simulink model "main"  (R2021a)
settings: Solver=ode113  StartTime=0.0  StopTime=300  RelTol=1e-13  AbsTol=1e-14
values from neighbouring files (symbols this model uses):
  Const = createSimulinkBus(Const_1)    [initializeData.m]
  Earth = createSimulinkBus(Earth_1)    [initializeData.m]
  Sensors = createSimulinkBus(Sensors_1)    [initializeData.m]
  Spacecraft = createSimulinkBus(Spacecraft_1)    [initializeData.m]
  totalTorque = [0 0 0 0.000704944678681 0.000834848489248 0.000628617928475 0.000704944678681 -0.000834848489248 -0.000628617928475 0.00140988935736 0 0 ... (48 elements, 3x16)]    [totalTorque.mat]
undefined symbols (not defined in the file or in its folder): initCond, torqueLookUpTable
libraries: simulink x22, SADlibrary x22, aerolibutil x20, vrlib x14, dspsrcs4 x12, sharedtransform x5, commfilt2 x3, dspfdesign x3, simulink_extras x2, sharedTrackingLibrary x2, dspmathops x1, sharedutil x1
(part 1 of 2)
settings Model: SimulationMode=rapid-accelerator  Creator=matteo  LastModifiedBy=matteo
settings SolverCC: ZeroCrossControl=EnableAll  ZeroCrossAlgorithm=Adaptive  AlgebraicLoopSolver=TrustRegion  DecoupledContinuousIntegration=on
settings DebuggingCC: ReadBeforeWriteMsg=DisableAll  WriteAfterWriteMsg=DisableAll  WriteAfterReadMsg=DisableAll  MultiTaskDSMMsg=none  SFMachineParentedDataDiag=warning
settings ModelReferenceCC: UpdateModelReferenceTargets=IfOutOfDate
settings SFSimCC: SFSimEcho=off
settings SimscapeCC: SimscapeNormalizeSystem=off

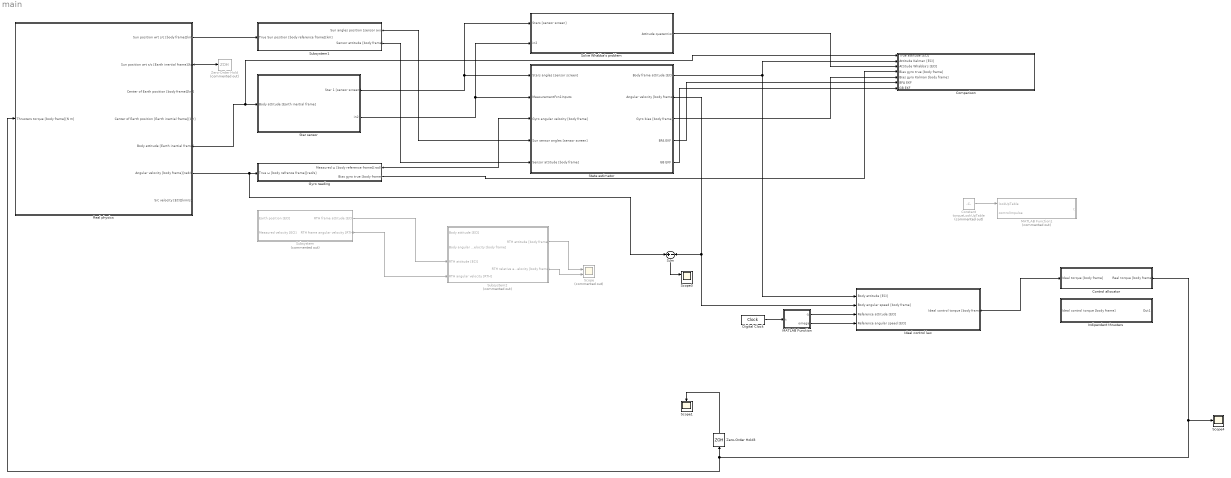
== system main ==
  Comparison : Subsystem
  Constant : Constant  Commented=on  Value=torqueLookUpTable
  Control allocator : Subsystem
  Digital Clock : DigitalClock  SampleTime=1/1000
  Gyro reading : Subsystem
  Ideal control law : Subsystem
  Indipendent thrusters : Subsystem
  MATLAB Function : MATLAB Function  TreatAsAtomicUnit=on
  MATLAB Function1 : MATLAB Function  Commented=on  TreatAsAtomicUnit=on
  Real physics : Subsystem
  Scope : Scope  Commented=on  NumInputPorts=2
  Scope1 : Scope
  Scope3 : Scope  NumInputPorts=2
  Scope4 : Scope
  Solve Whabba's problem : Subsystem
  Star sensor : Subsystem
  State estimator : Subsystem
  Subsystem : Subsystem  Commented=on
  Subsystem1 : Subsystem
  Subsystem2 : Subsystem  Commented=on
  Sum : Sum  Inputs=+-
  Zero-Order Hold : ZeroOrderHold  Commented=on  SampleTime=Sensors.sunSensorSamplingFreq
  Zero-Order Hold3 : ZeroOrderHold  SampleTime=.01
  wires:
  Real physics/6(Angular velocity [body frame][rad/s]) -> Sum/1, Gyro reading/1(True ω [body refrence frame][rad/s])
  Real physics/2(Sun position wrt s/c [Earth inertial frame][km]) -> Zero-Order Hold/1
  Real physics/1(Sun position wrt s/c [body frame][km]) -> Subsystem1/1(True Sun position [body reference frame][km])
  Subsystem/1(RTH frame attitude [ECI]) -> Subsystem2/3(RTH attitude [ECI])
  Subsystem/2("RTH frame angular velocity [RTH] ") -> Subsystem2/4(RTH angular velocity [RTH])
  Subsystem2/1(RTH attitude [body frame]) -> Scope/1
  Subsystem2/2(RTH relative angular velocity [body frame]) -> Scope/2
  Zero-Order Hold3/1 -> Scope1/1
  Real physics/5(Body attitude [Earth inertial frame]) -> Comparison/1(True attitude [ECI]), Star sensor/1(Body attitude [Earth inertial frame])
  Star sensor/1(Star 1 [sensor screen]) -> Solve Whabba's problem/1(Stars [sensor screen]), State estimator/1(Stars angles [sensor screen])
  Star sensor/2(in2) -> State estimator/2(MeasurementFcn1Inputs), Solve Whabba's problem/2(in2)
  Gyro reading/1(Measured ω [body reference frame][rad/s]) -> State estimator/3(Gyro angular velocity [body frame])
  State estimator/1(Body frame attitude [ECI]) -> Ideal control law/1(Body attitude [ECI]), Comparison/2(Attitude Kalman [ECI])
  Solve Whabba's problem/1(Attitude quaternion) -> Comparison/3(Attitude Whabba's [ECI])
  State estimator/2(Angular velocity [body frame]) -> Sum/2, Ideal control law/2(Body angular speed [body frame])
  Gyro reading/2(Bias gyro true [body frame]) -> Comparison/4(Bias gyro true [body frame])
  State estimator/3(Gyro bias [body frame]) -> Comparison/5(Bias gyro Kalman [body frame])
  Sum/1 -> Scope3/1
  MATLAB Function/1(q) -> Ideal control law/3(Reference attitude [ECI])
  MATLAB Function/2(omega) -> Ideal control law/4(Reference angular speed [ECI])
  State estimator/4(BFA EKF) -> Comparison/6(BFA EKF)
  State estimator/5(GB EKF) -> Comparison/7(GB EKF)
  Constant/1 -> MATLAB Function1/1(lookUpTable)
  Digital Clock/1 -> MATLAB Function/1(t)
  Control allocator/1(Real torque [body frame]) -> Real physics/1(Thrusters torque [body frame][N m]), Zero-Order Hold3/1, Scope4/1
  Subsystem1/1(Sun angles position [sensor axis]) -> State estimator/4(Sun sensor angles [sensor screen])
  Subsystem1/2(Sensor attitude [body frame]) -> State estimator/5(Sensor attitude [body frame])
  Ideal control law/1(Ideal control torque [body frame]) -> Control allocator/1(Ideal torque [body frame])

== system main/Comparison ==
  True attitude [ECI] : Inport
  Attitude Kalman [ECI] : Inport  Port=2
  Attitude Whabba's [ECI] : Inport  Port=3
  Bias gyro true [body frame] : Inport  Port=4
  Bias gyro Kalman [body frame] : Inport  Port=5
  BFA EKF : Inport  Port=6
  GB EKF : Inport  Port=7
  MATLAB Function : MATLAB Function  TreatAsAtomicUnit=on
  MATLAB Function1 : MATLAB Function  TreatAsAtomicUnit=on
  MATLAB Function2 : MATLAB Function  TreatAsAtomicUnit=on
  Quaternion Division1 : aerolibutil/Quaternion Division
      settings: SourceProductBaseCode=AE
  Quaternion Division2 : aerolibutil/Quaternion Division
      settings: SourceProductBaseCode=AE
  Quaternion Division3 : aerolibutil/Quaternion Division
      settings: SourceProductBaseCode=AE
  Scope : Scope  NumInputPorts=3
  Scope1 : Scope  NumInputPorts=3
  wires:
  True attitude [ECI]/1 -> Quaternion Division3/1, Quaternion Division1/1, Quaternion Division2/1
  Attitude Kalman [ECI]/1 -> Quaternion Division2/2
  Attitude Whabba's [ECI]/1 -> Quaternion Division1/2
  Quaternion Division2/1 -> MATLAB Function1/1(q)  "Kalman error"
  Bias gyro true [body frame]/1 -> Scope1/1
  Bias gyro Kalman [body frame]/1 -> Scope1/2
  MATLAB Function1/1(e) -> Scope/1  "Kalman error"
  MATLAB Function/1(e) -> Scope/2  "Whabba's error"
  Quaternion Division1/1 -> MATLAB Function/1(q)  "Whabba's error"
  BFA EKF/1 -> Quaternion Division3/2
  Quaternion Division3/1 -> MATLAB Function2/1(q)  "Whabba's error"
  MATLAB Function2/1(e) -> Scope/3  "Whabba's error"
  GB EKF/1 -> Scope1/3

== system main/Control allocator ==
  Ideal torque [body frame] : Inport
  Constant1 : Constant  Value=thrustersTorque'  VectorParams1D=off
  Demux3 : Demux  Outputs=3
  Gain18 : Gain
  Gain19 : Gain
  Gain5 : Gain  Gain=1/2
  Integrate and Dump4 : commfilt2/Integrate and Dump  obssamples=200  offsetsamples=0  nodump=off  roundingMode=Floor  overflowMode=off  outputDataTypeStr=Inherit: Same as accumulator  outputLastDataTypeStr=Inherit: Same as accumulator
  Integrate and Dump5 : commfilt2/Integrate and Dump  obssamples=200  offsetsamples=0  nodump=off  roundingMode=Floor  overflowMode=off  outputDataTypeStr=Inherit: Same as accumulator  outputLastDataTypeStr=Inherit: Same as accumulator
  Integrate and Dump6 : commfilt2/Integrate and Dump  obssamples=200  offsetsamples=0  nodump=off  roundingMode=Floor  overflowMode=off  outputDataTypeStr=Inherit: Same as accumulator  outputLastDataTypeStr=Inherit: Same as accumulator
  MATLAB Function3 : MATLAB Function  TreatAsAtomicUnit=on
  Mux2 : Mux  Inputs=3
  Subsystem3 : Subsystem
  Real torque [body frame] : Outport
  wires:
  Gain19/1 -> Real torque [body frame]/1
  Gain18/1 -> MATLAB Function3/1(cgtTorque)
  Integrate and Dump6/1 -> Mux2/1
  Demux3/2 -> Integrate and Dump4/1
  Gain5/1 -> MATLAB Function3/2(dGammaId)
  Constant1/1 -> Gain18/1
  MATLAB Function3/1(xOpt) -> Subsystem3/1(uTimes)
  Demux3/1 -> Integrate and Dump6/1
  Demux3/3 -> Integrate and Dump5/1
  Subsystem3/1(Real torque) -> Gain19/1
  Mux2/1 -> Gain5/1
  Integrate and Dump4/1 -> Mux2/2
  Ideal torque [body frame]/1 -> Demux3/1
  Integrate and Dump5/1 -> Mux2/3

== system main/Gyro reading ==
  True ω [body refrence frame][rad/s] : Inport
  Constant : Constant  Value=1e-3*randn(3,1)
  Cumulative Sum : dspmathops/Cumulative Sum  dim=Channels (running sum)  reset_popup=None  roundingMode=Floor  overflowMode=off  outputDataTypeStr=Inherit: Same as accumulator  outputMin=[]  outputMax=[]  outputLastDataTypeStr=Inherit: Same as accumulator
  Gain : Gain  Gain=sqrt(1/Sensors.gyroSamplingFreq)
  Random Source : dspsrcs4/Random Source  SrcType=Gaussian  NormMethod=Ziggurat  CltLength=12  MinVal=0  MaxVal=1  MeanVal=0  VarVal=Sensors.gyroCovariance  RepMode=Not repeatable  rawSeed=1  IsInherit=off  SampMode=Discrete  SampTime=1/Sensors.gyroSamplingFreq  SampFrame=3  DataType=Double  OutComplex=Real  OutputFrames=off
  Random Source1 : dspsrcs4/Random Source  SrcType=Gaussian  NormMethod=Ziggurat  CltLength=12  MinVal=0  MaxVal=1  MeanVal=0  VarVal=Sensors.gyroBiasInstability  RepMode=Not repeatable  rawSeed=1  IsInherit=off  SampMode=Discrete  SampTime=1/Sensors.gyroSamplingFreq  SampFrame=3  DataType=Double  OutComplex=Real  OutputFrames=off
  Sum : Sum  Inputs=|++
  Sum1 : Sum  Inputs=|++
  Sum2 : Sum  Inputs=|++
  Zero-Order Hold : ZeroOrderHold  SampleTime=1/Sensors.gyroSamplingFreq
  Measured ω [body reference frame][rad/s] : Outport
  Bias gyro true [body frame] : Outport  Port=2
  wires:
  Sum2/1 -> Measured ω [body reference frame][rad/s]/1
  True ω [body refrence frame][rad/s]/1 -> Zero-Order Hold/1
  Cumulative Sum/1 -> Sum1/2
  Gain/1 -> Cumulative Sum/1
  Random Source1/1 -> Gain/1
  Constant/1 -> Sum1/1
  Zero-Order Hold/1 -> Sum/1
  Random Source/1 -> Sum/2
  Sum/1 -> Sum2/1
  Sum1/1 -> Bias gyro true [body frame]/1, Sum2/2

== system main/Ideal control law ==
  note: $q_e := q_{B/R} = q_{B/N} \otimes q_{R/N}^{-1}$
  Body attitude [ECI] : Inport
  Body angular speed [body frame] : Inport  Port=2
  Reference attitude [ECI] : Inport  Port=3
  Reference angular speed [ECI] : Inport  Port=4
  Constant : Constant  Value=Spacecraft.baricentricInertia
  Constant1 : Constant  Value=totalTorque
  MATLAB Function : MATLAB Function  TreatAsAtomicUnit=on
  MATLAB Function1 : MATLAB Function  TreatAsAtomicUnit=on
  MATLAB Function2 : MATLAB Function  TreatAsAtomicUnit=on
  Quaternion Division : aerolibutil/Quaternion Division
      settings: SourceProductBaseCode=AE
  Quaternion Rotation : aerolibutil/Quaternion Rotation
  Scope : Scope  NumInputPorts=4
  Scope1 : Scope
  Scope2 : Scope
  Sum : Sum  Inputs=|+-
  Ideal control torque [body frame] : Outport
  wires:
  Quaternion Division/1 -> MATLAB Function1/1(q), MATLAB Function2/5(qErr), MATLAB Function/4(qErr), Scope/1  "Attitude error"
  Reference angular speed [ECI]/1 -> Quaternion Rotation/2
  Quaternion Rotation/1 -> Sum/2  "Reference angular speed [body frame]"
  Body angular speed [body frame]/1 -> MATLAB Function2/3(omegaBody), MATLAB Function/2(omegaBody), Sum/1
  Sum/1 -> Scope1/1, MATLAB Function2/4(omegaErr), MATLAB Function/3(omegaErr)  "Angular speed error [body frame]"
  Constant/1 -> MATLAB Function/1(J), MATLAB Function2/1(J)
  Reference attitude [ECI]/1 -> Scope/4, Quaternion Division/2
  Body attitude [ECI]/1 -> Scope/3, Quaternion Division/1, Quaternion Rotation/1
  MATLAB Function1/1(e) -> Scope/2
  Constant1/1 -> MATLAB Function2/2(torque)
  MATLAB Function2/2(VdotMin) -> Scope2/1
  MATLAB Function/1(u) -> Ideal control torque [body frame]/1

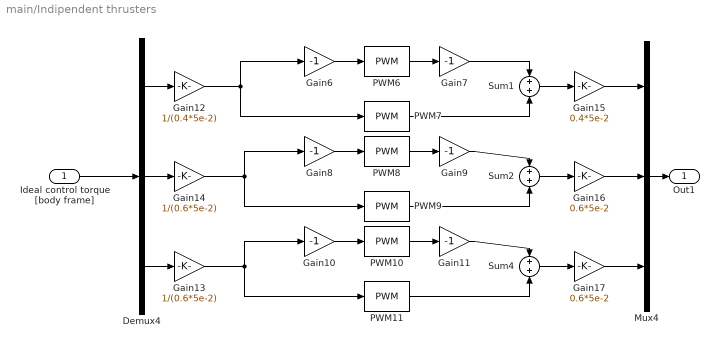
== system main/Indipendent thrusters ==
  Ideal control torque [body frame] : Inport
  Demux4 : Demux  Outputs=3
  Gain{6..11} (6 alike) : Gain  Gain=-1
  Gain12 : Gain  Gain=1/(0.4*5e-2)
  Gain13 : Gain  Gain=1/(0.6*5e-2)
  Gain14 : Gain  Gain=1/(0.6*5e-2)
  Gain15 : Gain  Gain=0.4*5e-2
  Gain16 : Gain  Gain=0.6*5e-2
  Gain17 : Gain  Gain=0.6*5e-2
  Mux4 : Mux  Inputs=3
  PWM{6..11} (6 alike) : simulink/Discontinuities/PWM  DisableCoverage=on  Period=0.5  DisallowZeroDutyCycle=off  RunAtFixedTimeIntervals=on  SampleTime=1/Sensors.gyroSamplingFreq
  Sum1 : Sum
  Sum2 : Sum
  Sum4 : Sum
  Out1 : Outport
  wires:
  PWM8/1 -> Gain9/1
  Mux4/1 -> Out1/1
  PWM11/1 -> Sum4/2
  Gain11/1 -> Sum4/1
  PWM6/1 -> Gain7/1
  Sum2/1 -> Gain16/1
  PWM10/1 -> Gain11/1
  Gain12/1 -> PWM7/1, Gain6/1
  Gain17/1 -> Mux4/3
  PWM7/1 -> Sum1/2
  Gain6/1 -> PWM6/1
  Gain16/1 -> Mux4/2
  Gain9/1 -> Sum2/1
  Gain14/1 -> PWM9/1, Gain8/1
  Demux4/1 -> Gain12/1
  Gain10/1 -> PWM10/1
  Gain13/1 -> PWM11/1, Gain10/1
  Demux4/2 -> Gain14/1
  Sum4/1 -> Gain17/1
  Ideal control torque [body frame]/1 -> Demux4/1
  Sum1/1 -> Gain15/1
  Gain8/1 -> PWM8/1
  Gain15/1 -> Mux4/1
  Demux4/3 -> Gain13/1
  PWM9/1 -> Sum2/2
  Gain7/1 -> Sum1/1

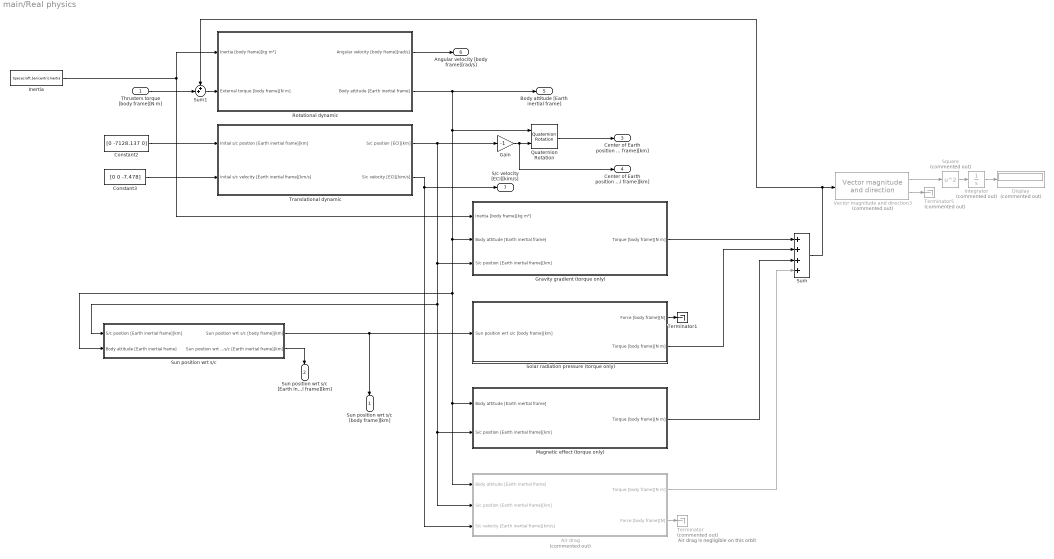
== system main/Real physics ==
  note: Air drag is negligible on this orbit
  Thrusters torque [body frame][N m] : Inport  Unit=N*m
  Air drag : Subsystem  Commented=on
  Constant2 : Constant  Value=[0 -7128.137 0]
  Constant3 : Constant  Value=[0 0 -7.478]
  Display : Display  Commented=on
  Gain : Gain  Gain=-1
  Gravity gradient (torque only) : Subsystem
      settings: PortSchema="{\"entries\":[{\"content\":{\"sides\":[{\"content\":{\"connectorIds\":[\"Out1\"]},\"type\":\"ConnectorPlacement.EquallySpacedRectSide\",\"uuid\":\"f1f9fb06-69b8-4265-b1e3-1bc99765f445\"},{\"content\":{\"connectorIds\":[\"In1\",\"In2\",\"In3\"],\"side\":\"RIGHT\"},\"type\":\"ConnectorPlacement.EquallySpacedRectSide\",\"uuid\":\"95872401-8fe8-493a-a743-72ee2e043305\"},{\"content\":{\"connectorIds\":[],\"side\":\"TOP\"},\"type\":\"ConnectorPlacement.EquallySpacedRectSide\",\"uuid\":\"a2f933f3-d116-4556-b216-8e543aff18f5\"},{\"content\":{\"connectorIds\":[],\"side\":\"HIDDEN\"},\"type\":\"ConnectorPlacement.EquallySpacedRectSide\",\"uuid\":\"93d45030-e624-494e-a335-b0ea445a7c18\"}]},\"type\":\"ConnectorPlacement.EquallySpacedConnector\",\"uuid\":\"bbb7bc93-29be-48e8-9ed7-f6b41cc2b7e1\"}],\"packageUris\":[\"http://schema.mathworks.com/mf0/Connector/R2020b\"],\"version\":\"1.0\"}"
  Inertia : Constant  Value=Spacecraft.baricentricInertia
  Integrator : Integrator  Commented=on
  Magnetic effect (torque only) : Subsystem
  Quaternion Rotation : aerolibutil/Quaternion Rotation
  Rotational dynamic : Subsystem
  Solar radiation pressure (torque only) : Subsystem
  Square : Math  Commented=on  Operator=square  SaturateOnIntegerOverflow=on
  Sum : Sum  Inputs=++++
  Sum1 : Sum  Inputs=++|
  Sun position wrt s/c : Subsystem
  Terminator : Terminator  Commented=on
  Terminator1 : Terminator
  Terminator5 : Terminator  Commented=on
  Translational dynamic : Subsystem
  Vector magnitude and direction3 : SADlibrary/Vector magnitude and direction  Commented=on  SystemSampleTime=-1  VariantActivationTime=update diagram  Latency=0  AutoFrameSizeCalculation=off
  Sun position wrt s/c [body frame][km] : Outport  OutDataTypeStr=double  Unit=km
  Sun position wrt s/c [Earth inertial frame][km] : Outport  Port=2
  Center of Earth position [body frame][km] : Outport  Port=3
  Center of Earth position [Earth inertial frame][km] : Outport  Port=4
  Body attitude [Earth inertial frame] : Outport  Port=5
  Angular velocity [body frame][rad/s] : Outport  Port=6
  S/c velocity [ECI][kim/s] : Outport  Port=7
  wires:
  Inertia/1 -> Gravity gradient (torque only)/1(Inertia [body frame][kg m²]), Rotational dynamic/1(Inertia [body frame][kg m²])
  Rotational dynamic/1(Angular velocity [body frame][rad/s]) -> Angular velocity [body frame][rad/s]/1
  Constant2/1 -> Translational dynamic/1(Initial s/c position [Earth inertial frame][km])
  Constant3/1 -> Translational dynamic/2(Initial s/c velocity [Earth inertial frame][km/s])
  Rotational dynamic/2(Body attitude [Earth inertial frame]) -> Body attitude [Earth inertial frame]/1, Quaternion Rotation/1, Air drag/1(Body attitude [Earth inertial frame]), Magnetic effect (torque only)/1(Body attitude [Earth inertial frame]), Sun position wrt s/c/2(Body attitude [Earth inertial frame]), Gravity gradient (torque only)/2(Body attitude [Earth inertial frame])
  Translational dynamic/1(S/c position [ECI][km]) -> Gain/1, Gravity gradient (torque only)/3(S/c position [Earth inertial frame][km]), Sun position wrt s/c/1(S/c position [Earth inertial frame][km]), Air drag/2(S/c position [Earth inertial frame][km]), Magnetic effect (torque only)/2(S/c position [Earth inertial frame][km])
  Sum/1 -> Sum1/1, Vector magnitude and direction3/1
  Air drag/2(Force [body frame][N]) -> Terminator/1
  Solar radiation pressure (torque only)/1(Force [body frame][N]) -> Terminator1/1
  Sun position wrt s/c/1(Sun position wrt s/c [body frame][km]) -> Solar radiation pressure (torque only)/1(Sun position wrt s/c [body frame][km]), Sun position wrt s/c [body frame][km]/1
  Solar radiation pressure (torque only)/2(Torque [body frame][N m]) -> Sum/2
  Magnetic effect (torque only)/1(Torque [body frame][N m]) -> Sum/3
  Air drag/1(Torque [body frame][N m]) -> Sum/4
  Gravity gradient (torque only)/1(Torque [body frame][N m]) -> Sum/1
  Gain/1 -> Center of Earth position [Earth inertial frame][km]/1, Quaternion Rotation/2
  Quaternion Rotation/1 -> Center of Earth position [body frame][km]/1
  Sun position wrt s/c/2(Sun position wrt s/c [Earth inertial frame][km]) -> Sun position wrt s/c [Earth inertial frame][km]/1
  Thrusters torque [body frame][N m]/1 -> Sum1/2
  Sum1/1 -> Rotational dynamic/2(External torque [body frame][N m])
  Vector magnitude and direction3/1 -> Square/1
  Vector magnitude and direction3/2 -> Terminator5/1
  Square/1 -> Integrator/1
  Integrator/1 -> Display/1
  Translational dynamic/2(S/c velocity [ECI][kim/s]) -> S/c velocity [ECI][kim/s]/1, Air drag/3(S/c velocity [Earth inertial frame][km/s])

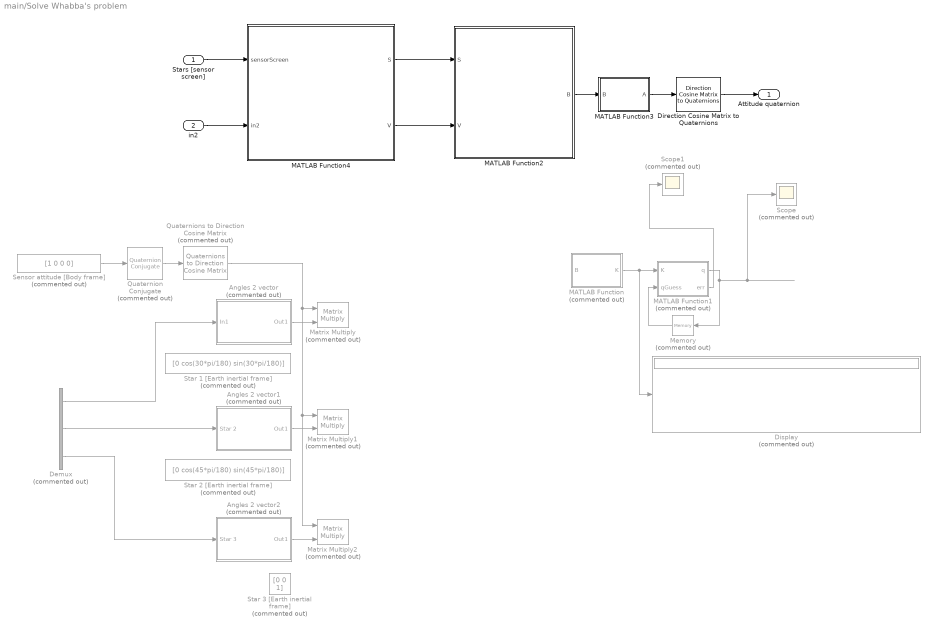
== system main/Solve Whabba's problem ==
  Stars [sensor screen] : Inport
  in2 : Inport  Port=2
  Angles 2 vector : Subsystem  Commented=on
  Angles 2 vector1 : Subsystem  Commented=on
  Angles 2 vector2 : Subsystem  Commented=on
  Demux : Demux  Commented=on  Outputs=3
  Direction Cosine Matrix to Quaternions : sharedtransform/Direction Cosine Matrix  to Quaternions  aMode=0  action=None  tolerance=eps(2)
      settings: SourceProductBaseCode=AE,PW,DR,MT,UV,VE
  Display : Display  Commented=on
  MATLAB Function : MATLAB Function  Commented=on  TreatAsAtomicUnit=on
  MATLAB Function1 : MATLAB Function  Commented=on  TreatAsAtomicUnit=on
  MATLAB Function2 : MATLAB Function  TreatAsAtomicUnit=on
  MATLAB Function3 : MATLAB Function  TreatAsAtomicUnit=on
  MATLAB Function4 : MATLAB Function  TreatAsAtomicUnit=on
  Matrix Multiply : Product  Commented=on  Multiplication=Matrix(*)
  Matrix Multiply1 : Product  Commented=on  Multiplication=Matrix(*)
  Matrix Multiply2 : Product  Commented=on  Multiplication=Matrix(*)
  Memory : Memory  Commented=on  InitialCondition=[1 0 0 0]
  Quaternion Conjugate : aerolibutil/Quaternion Conjugate  Commented=on
      settings: SourceProductBaseCode=AE
  Quaternions to Direction Cosine Matrix : sharedtransform/Quaternions to  Direction Cosine Matrix  Commented=on  aMode=aMode
      settings: SourceProductBaseCode=AE,PW,DR,MT,UV,VE
  Scope : Scope  Commented=on
  Scope1 : Scope  Commented=on
  Sensor attitude [Body frame] : Constant  Commented=on  Value=[1 0 0 0]
  Star 1 [Earth inertial frame] : Constant  Commented=on  Value=[0 cos(30*pi/180) sin(30*pi/180)]
  Star 2 [Earth inertial frame] : Constant  Commented=on  Value=[0 cos(45*pi/180) sin(45*pi/180)]
  Star 3 [Earth inertial frame] : Constant  Commented=on  Value=[0 0 1]
  Attitude quaternion : Outport
  wires:
  Demux/1 -> Angles 2 vector/1(In1)
  Demux/2 -> Angles 2 vector1/1(Star 2)
  Demux/3 -> Angles 2 vector2/1(Star 3)
  Angles 2 vector/1(Out1) -> Matrix Multiply/2
  MATLAB Function2/1(B) -> MATLAB Function3/1(B)
  MATLAB Function/1(K) -> Display/1, MATLAB Function1/1(K)
  MATLAB Function1/1(q) -> Memory/1, Scope/1
  Sensor attitude [Body frame]/1 -> Quaternion Conjugate/1
  Quaternion Conjugate/1 -> Quaternions to Direction Cosine Matrix/1
  Quaternions to Direction Cosine Matrix/1 -> Matrix Multiply2/1, Matrix Multiply1/1, Matrix Multiply/1
  Angles 2 vector2/1(Out1) -> Matrix Multiply2/2
  Angles 2 vector1/1(Out1) -> Matrix Multiply1/2
  Memory/1 -> MATLAB Function1/2(qGuess)
  MATLAB Function1/2(err) -> Scope1/1
  MATLAB Function3/1(A) -> Direction Cosine Matrix to Quaternions/1
  Direction Cosine Matrix to Quaternions/1 -> Attitude quaternion/1
  MATLAB Function4/1(S) -> MATLAB Function2/1(S)
  MATLAB Function4/2(V) -> MATLAB Function2/2(V)
  Stars [sensor screen]/1 -> MATLAB Function4/1(sensorScreen)
  in2/1 -> MATLAB Function4/2(in2)

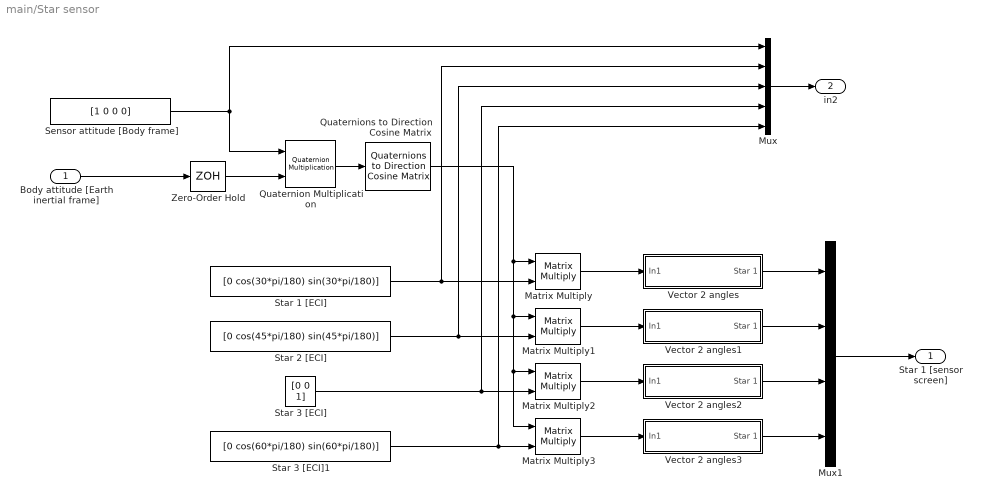
== system main/Star sensor ==
  Body attitude [Earth inertial frame] : Inport
  Matrix Multiply{,1..3} (4 alike) : Product  Multiplication=Matrix(*)
  Mux : Mux  Inputs=5
  Mux1 : Mux
  Quaternion Multiplication : aerolibutil/Quaternion Multiplication
  Quaternions to Direction Cosine Matrix : sharedtransform/Quaternions to  Direction Cosine Matrix  aMode=aMode
      settings: SourceProductBaseCode=AE,PW,DR,MT,UV,VE
  Sensor attitude [Body frame] : Constant  Value=[1 0 0 0]
  Star 1 [ECI] : Constant  Value=[0 cos(30*pi/180) sin(30*pi/180)]
  Star 2 [ECI] : Constant  Value=[0 cos(45*pi/180) sin(45*pi/180)]
  Star 3 [ECI] : Constant  Value=[0 0 1]
  Star 3 [ECI]1 : Constant  Value=[0 cos(60*pi/180) sin(60*pi/180)]
  Vector 2 angles : Subsystem
  Vector 2 angles1 : Subsystem
  Vector 2 angles2 : Subsystem
  Vector 2 angles3 : Subsystem
  Zero-Order Hold : ZeroOrderHold  SampleTime=1/Sensors.starTrackerSamplingFreq
  Star 1 [sensor screen] : Outport
  in2 : Outport  Port=2
  wires:
  Body attitude [Earth inertial frame]/1 -> Zero-Order Hold/1
  Sensor attitude [Body frame]/1 -> Mux/1, Quaternion Multiplication/1
  Quaternion Multiplication/1 -> Quaternions to Direction Cosine Matrix/1
  Star 1 [ECI]/1 -> Matrix Multiply/2, Mux/2
  Star 2 [ECI]/1 -> Mux/3, Matrix Multiply1/2
  Star 3 [ECI]/1 -> Mux/4, Matrix Multiply2/2
  Quaternions to Direction Cosine Matrix/1 -> Matrix Multiply3/1, Matrix Multiply2/1, Matrix Multiply1/1, Matrix Multiply/1
  Matrix Multiply/1 -> Vector 2 angles/1(In1)
  Matrix Multiply2/1 -> Vector 2 angles2/1(In1)
  Matrix Multiply1/1 -> Vector 2 angles1/1(In1)
  Vector 2 angles1/1(Star 1) -> Mux1/2
  Vector 2 angles2/1(Star 1) -> Mux1/3
  Vector 2 angles/1(Star 1) -> Mux1/1
  Mux/1 -> in2/1
  Zero-Order Hold/1 -> Quaternion Multiplication/2
  Mux1/1 -> Star 1 [sensor screen]/1
  Star 3 [ECI]1/1 -> Mux/5, Matrix Multiply3/2
  Matrix Multiply3/1 -> Vector 2 angles3/1(In1)
  Vector 2 angles3/1(Star 1) -> Mux1/4

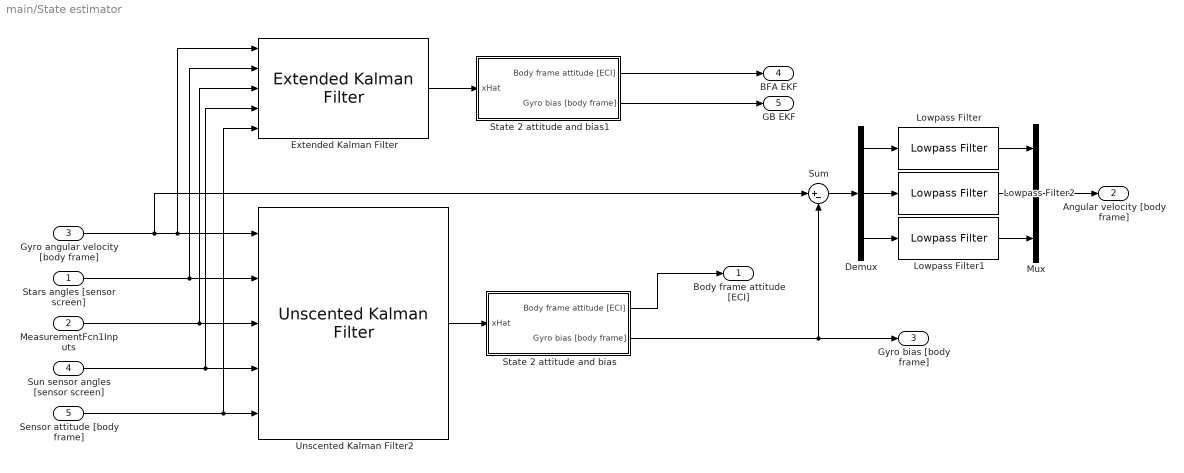
== system main/State estimator ==
  Stars angles [sensor screen] : Inport
  MeasurementFcn1Inputs : Inport  Port=2
  Gyro angular velocity [body frame] : Inport  Port=3
  Sun sensor angles [sensor screen] : Inport  Port=4
  Sensor attitude [body frame] : Inport  Port=5
  Demux : Demux  Outputs=3
  Extended Kalman Filter : sharedTrackingLibrary/Extended Kalman Filter  StateTransitionFcn=statePropagation  HasStateTransitionJacobianFcn=off  HasAdditiveProcessNoise=Nonadditive  ProcessNoise=diag([Sensors.gyroCovariance * [1 1 1], Sensors.gyroBiasInstability * [1 1 1]])  HasTimeVaryingProcessNoise=off  HasStateTransitionFcnExtraArgument=1  InitialState=[Spacecraft.initialAttitude' 0 0 0]'  InitialStateCovariance=1e-6*eye(7)  MeasurementFcn1=simulateStarSensor  HasMeasurementJacobianFcn1=off  HasMeasurementEnablePort1=off  HasAdditiveMeasurementNoise1=Additive  MeasurementNoise1=Sensors.starTrackerCovariance*eye(8)  HasTimeVaryingMeasurementNoise1=off  HasMeasurementFcnExtraArgument1=1  MeasurementFcn2=simulateSunSensor  HasMeasurementJacobianFcn2=off  HasMeasurementEnablePort2=off  HasAdditiveMeasurementNoise2=Additive  MeasurementNoise2=(.1*pi/180)^2*eye(2)  HasTimeVaryingMeasurementNoise2=off  HasMeasurementFcnExtraArgument2=1  MeasurementFcn3=myMeasurementFcn  HasMeasurementJacobianFcn3=off  HasMeasurementEnablePort3=off  HasAdditiveMeasurementNoise3=Additive  MeasurementNoise3=1  HasTimeVaryingMeasurementNoise3=off  HasMeasurementFcnExtraArgument3=0  MeasurementFcn4=myMeasurementFcn  HasMeasurementJacobianFcn4=off  HasMeasurementEnablePort4=off  HasAdditiveMeasurementNoise4=Additive  MeasurementNoise4=1  HasTimeVaryingMeasurementNoise4=off  HasMeasurementFcnExtraArgument4=0  MeasurementFcn5=myMeasurementFcn  HasMeasurementJacobianFcn5=off  HasMeasurementEnablePort5=off  HasAdditiveMeasurementNoise5=Additive  MeasurementNoise5=1  HasTimeVaryingMeasurementNoise5=off  HasMeasurementFcnExtraArgument5=0  EnableMultirate=on  StateTransitionFcnSampleTime=1/Sensors.gyroSamplingFreq  MeasurementFcn1SampleTime=1/Sensors.starTrackerSamplingFreq  MeasurementFcn2SampleTime=1  MeasurementFcn3SampleTime=1  MeasurementFcn4SampleTime=1  MeasurementFcn5SampleTime=1  UseCurrentEstimator=on  OutputStateCovariance=off  DataType=double  SampleTime=1  NumberOfMeasurements=2
      settings: SourceProductBaseCode=CT,DR,TF,ID,LP,NV,AR,RO,RR,UV,VE
  Lowpass Filter : dspfdesign/Lowpass Filter  FilterType=FIR  DesignForMinimumOrder=on  FilterOrder=50  PassbandFrequency=20  StopbandFrequency=40  PassbandRipple=0.0001  StopbandAttenuation=80  InheritSampleRate=off  SampleRate=100  SimulateUsing=Interpreted execution  roundingMode=Floor  coeffsDataTypeStr=fixdt(1,16)
  Lowpass Filter1 : dspfdesign/Lowpass Filter  FilterType=FIR  DesignForMinimumOrder=on  FilterOrder=50  PassbandFrequency=20  StopbandFrequency=40  PassbandRipple=0.0001  StopbandAttenuation=80  InheritSampleRate=off  SampleRate=100  SimulateUsing=Interpreted execution  roundingMode=Floor  coeffsDataTypeStr=fixdt(1,16)
  Lowpass Filter2 : dspfdesign/Lowpass Filter  FilterType=FIR  DesignForMinimumOrder=on  FilterOrder=50  PassbandFrequency=20  StopbandFrequency=40  PassbandRipple=0.0001  StopbandAttenuation=80  InheritSampleRate=off  SampleRate=100  SimulateUsing=Interpreted execution  roundingMode=Floor  coeffsDataTypeStr=fixdt(1,16)
  Mux : Mux  Inputs=3
  State 2 attitude and bias : Subsystem
  State 2 attitude and bias1 : Subsystem
  Sum : Sum  Inputs=|+-
  Unscented Kalman Filter2 : sharedTrackingLibrary/Unscented Kalman Filter  StateTransitionFcn=statePropagation  HasAdditiveProcessNoise=Nonadditive  ProcessNoise=diag([Sensors.gyroCovariance * [1 1 1], Sensors.gyroBiasInstability * [1 1 1]])  HasTimeVaryingProcessNoise=off  HasStateTransitionFcnExtraArgument=1  InitialState=[Spacecraft.initialAttitude' 0 0 0]'  InitialStateCovariance=1e-6*eye(7)  Alpha=1e-3  Beta=2  Kappa=0  MeasurementFcn1=simulateStarSensor  HasMeasurementEnablePort1=off  HasAdditiveMeasurementNoise1=Additive  MeasurementNoise1=Sensors.starTrackerCovariance*eye(8)  HasTimeVaryingMeasurementNoise1=off  HasMeasurementFcnExtraArgument1=1  MeasurementFcn2=simulateSunSensor  HasMeasurementEnablePort2=off  HasAdditiveMeasurementNoise2=Additive  MeasurementNoise2=(.1*pi/180)^2*eye(2)  HasTimeVaryingMeasurementNoise2=off  HasMeasurementFcnExtraArgument2=1  MeasurementFcn3=simulateSunSensor  HasMeasurementEnablePort3=off  HasAdditiveMeasurementNoise3=Additive  MeasurementNoise3=(.1*pi/180)^2*eye(2)  HasTimeVaryingMeasurementNoise3=off  HasMeasurementFcnExtraArgument3=1  MeasurementFcn4=myMeasurementFcn  HasMeasurementEnablePort4=off  HasAdditiveMeasurementNoise4=Additive  MeasurementNoise4=1  HasTimeVaryingMeasurementNoise4=off  HasMeasurementFcnExtraArgument4=0  MeasurementFcn5=myMeasurementFcn  HasMeasurementEnablePort5=off  HasAdditiveMeasurementNoise5=Additive  MeasurementNoise5=1  HasTimeVaryingMeasurementNoise5=off  HasMeasurementFcnExtraArgument5=0  EnableMultirate=on  StateTransitionFcnSampleTime=1/Sensors.gyroSamplingFreq  MeasurementFcn1SampleTime=1/Sensors.starTrackerSamplingFreq  MeasurementFcn2SampleTime=Sensors.sunSensorSamplingFreq  MeasurementFcn3SampleTime=Sensors.sunSensorSamplingFreq  MeasurementFcn4SampleTime=1  MeasurementFcn5SampleTime=1  UseCurrentEstimator=on  OutputStateCovariance=off  DataType=double  SampleTime=0.01  NumberOfMeasurements=2
      settings: SourceProductBaseCode=CT,DR,TF,ID,LP,NV,AR,RO,RR,UV,VE
  Body frame attitude [ECI] : Outport
  Angular velocity [body frame] : Outport  Port=2
  Gyro bias [body frame] : Outport  Port=3
  BFA EKF : Outport  Port=4
  GB EKF : Outport  Port=5
  wires:
  MeasurementFcn1Inputs/1 -> Extended Kalman Filter/3, Unscented Kalman Filter2/3
  State 2 attitude and bias/2(Gyro bias [body frame]) -> Gyro bias [body frame]/1, Sum/2
  State 2 attitude and bias/1(Body frame attitude [ECI]) -> Body frame attitude [ECI]/1
  Unscented Kalman Filter2/1 -> State 2 attitude and bias/1(xHat)
  Stars angles [sensor screen]/1 -> Unscented Kalman Filter2/2, Extended Kalman Filter/2
  Demux/1 -> Lowpass Filter/1
  Demux/2 -> Lowpass Filter2/1
  Demux/3 -> Lowpass Filter1/1
  Lowpass Filter/1 -> Mux/1
  Lowpass Filter1/1 -> Mux/3
  Lowpass Filter2/1 -> Mux/2
  Sum/1 -> Demux/1
  Mux/1 -> Angular velocity [body frame]/1
  Gyro angular velocity [body frame]/1 -> Unscented Kalman Filter2/1, Extended Kalman Filter/1, Sum/1
  Extended Kalman Filter/1 -> State 2 attitude and bias1/1(xHat)
  State 2 attitude and bias1/1(Body frame attitude [ECI]) -> BFA EKF/1
  State 2 attitude and bias1/2(Gyro bias [body frame]) -> GB EKF/1
  Sun sensor angles [sensor screen]/1 -> Extended Kalman Filter/4, Unscented Kalman Filter2/4
  Sensor attitude [body frame]/1 -> Extended Kalman Filter/5, Unscented Kalman Filter2/5

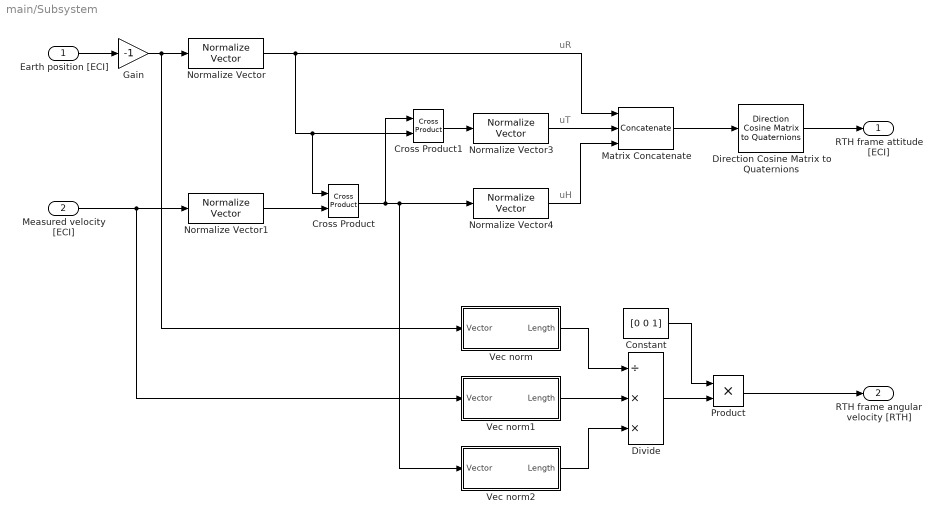
== system main/Subsystem ==
  note: uR
  note: uT
  note: uH
  Earth position [ECI] : Inport
  Measured velocity [ECI] : Inport  Port=2
  Constant : Constant  Value=[0 0 1]
  Cross Product : vrlib/Utilities/Cross Product
  Cross Product1 : vrlib/Utilities/Cross Product
  Direction Cosine Matrix to Quaternions : sharedtransform/Direction Cosine Matrix  to Quaternions  aMode=0  action=None  tolerance=eps(2)
      settings: SourceProductBaseCode=AE,PW,DR,MT,UV,VE
  Divide : Product  Inputs=/**
  Gain : Gain  Gain=-1
  Matrix Concatenate : Concatenate  NumInputs=3  Mode=Multidimensional array  ConcatenateDimension=2
  Normalize Vector{,1,3..4} (4 alike) : vrlib/Utilities/Normalize Vector  maxzero=0
  Product : Product
  Vec norm : Subsystem
  Vec norm1 : Subsystem
  Vec norm2 : Subsystem
  RTH frame attitude [ECI] : Outport
  "RTH frame angular velocity [RTH] " : Outport  Port=2
  wires:
  Matrix Concatenate/1 -> Direction Cosine Matrix to Quaternions/1
  Direction Cosine Matrix to Quaternions/1 -> RTH frame attitude [ECI]/1
  Earth position [ECI]/1 -> Gain/1
  Cross Product/1 -> Vec norm2/1(Vector), Normalize Vector4/1, Cross Product1/1
  Normalize Vector/1 -> Matrix Concatenate/1, Cross Product/1, Cross Product1/2
  Normalize Vector4/1 -> Matrix Concatenate/3
  Normalize Vector3/1 -> Matrix Concatenate/2
  Measured velocity [ECI]/1 -> Vec norm1/1(Vector), Normalize Vector1/1
  Cross Product1/1 -> Normalize Vector3/1
  Vec norm/1(Length) -> Divide/1
  Vec norm1/1(Length) -> Divide/2
  Vec norm2/1(Length) -> Divide/3
  Divide/1 -> Product/2
  Product/1 -> "RTH frame angular velocity [RTH] "/1
  Normalize Vector1/1 -> Cross Product/2
  Gain/1 -> Normalize Vector/1, Vec norm/1(Vector)
  Constant/1 -> Product/1

== system main/Subsystem1 ==
  True Sun position [body reference frame][km] : Inport
  MATLAB Function1 : MATLAB Function  TreatAsAtomicUnit=on
  Sun sensor reading1 : Subsystem
  Sun sensor reading2 : Subsystem
  Sun sensor reading3 : Subsystem
  Sun sensor reading4 : Subsystem
  Sun sensor reading5 : Subsystem
  Sun sensor reading6 : Subsystem
  Sun angles position [sensor axis] : Outport  PortDimensions=2
  Sensor attitude [body frame] : Outport  Port=2  PortDimensions=4
  wires:
  True Sun position [body reference frame][km]/1 -> Sun sensor reading3/1(True Sun position [body reference frame][km]), Sun sensor reading1/1(True Sun position [body reference frame][km]), Sun sensor reading2/1(True Sun position [body reference frame][km]), Sun sensor reading6/1(True Sun position [body reference frame][km]), Sun sensor reading5/1(True Sun position [body reference frame][km]), Sun sensor reading4/1(True Sun position [body reference frame][km])
  MATLAB Function1/2(sensAtt) -> Sensor attitude [body frame]/1
  Sun sensor reading2/1(Sun angles position [sensor axis]) -> MATLAB Function1/2(s2)
  Sun sensor reading1/1(Sun angles position [sensor axis]) -> MATLAB Function1/1(s1)
  Sun sensor reading3/1(Sun angles position [sensor axis]) -> MATLAB Function1/3(s3)
  Sun sensor reading4/1(Sun angles position [sensor axis]) -> MATLAB Function1/4(s4)
  Sun sensor reading5/1(Sun angles position [sensor axis]) -> MATLAB Function1/5(s5)
  Sun sensor reading6/1(Sun angles position [sensor axis]) -> MATLAB Function1/6(s6)
  MATLAB Function1/1(s) -> Sun angles position [sensor axis]/1

== system main/Subsystem2 ==
  Body attitude [ECI] : Inport
  Body angular velocity [body frame] : Inport  Port=2
  RTH attitude [ECI] : Inport  Port=3
  RTH angular velocity [RTH] : Inport  Port=4
  Quaternion Conjugate : aerolibutil/Quaternion Conjugate
      settings: SourceProductBaseCode=AE
  Quaternion Multiplication : aerolibutil/Quaternion Multiplication
  Quaternion Rotation : aerolibutil/Quaternion Rotation
  Sum1 : Sum  Inputs=+-
  RTH attitude [body frame] : Outport
  RTH relative angular velocity [body frame] : Outport  Port=2
  wires:
  Sum1/1 -> RTH relative angular velocity [body frame]/1
  Body angular velocity [body frame]/1 -> Sum1/2
  RTH attitude [ECI]/1 -> Quaternion Multiplication/1
  RTH angular velocity [RTH]/1 -> Quaternion Rotation/2
  Body attitude [ECI]/1 -> Quaternion Conjugate/1
  Quaternion Rotation/1 -> Sum1/1
  Quaternion Multiplication/1 -> Quaternion Rotation/1, RTH attitude [body frame]/1
  Quaternion Conjugate/1 -> Quaternion Multiplication/2

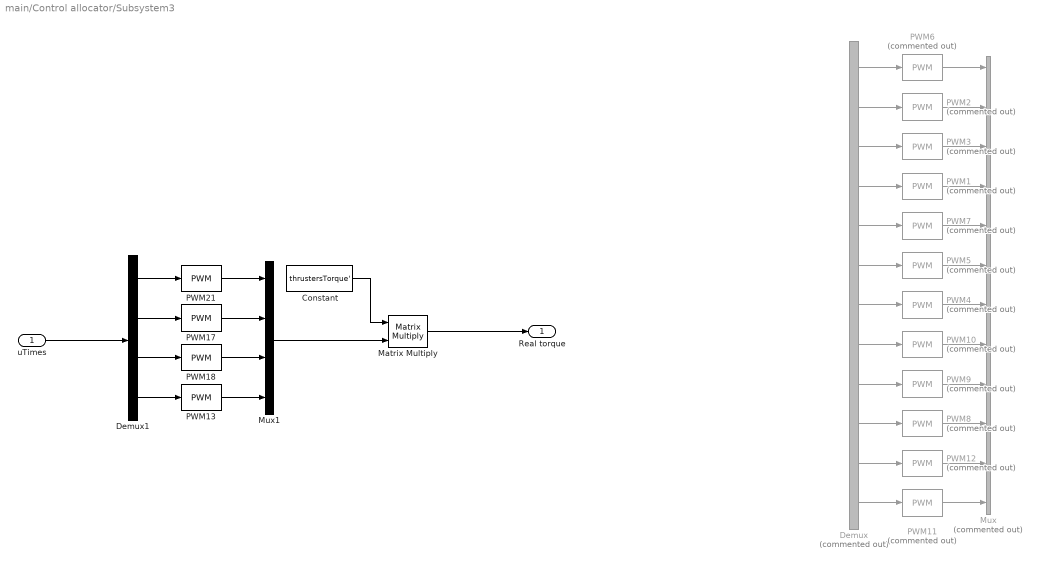
== system main/Control allocator/Subsystem3 ==
  uTimes : Inport
  Constant : Constant  Value=thrustersTorque'  VectorParams1D=off
  Demux : Demux  Commented=on  Outputs=12
  Demux1 : Demux
  Matrix Multiply : Product  Multiplication=Matrix(*)
  Mux : Mux  Commented=on  Inputs=12
  Mux1 : Mux
  PWM{1..12} (12 alike) : simulink/Discontinuities/PWM  Commented=on  DisableCoverage=on  Period=0.2  DisallowZeroDutyCycle=off  RunAtFixedTimeIntervals=on  SampleTime=0.02
  PWM{13,17..18,21} (4 alike) : simulink/Discontinuities/PWM  DisableCoverage=on  Period=0.2  DisallowZeroDutyCycle=off  RunAtFixedTimeIntervals=on  SampleTime=0.02
  Real torque : Outport
  wires:
  Demux/1 -> PWM6/1
  Demux/2 -> PWM2/1
  Demux/3 -> PWM3/1
  Demux/4 -> PWM1/1
  Demux/5 -> PWM7/1
  Demux/6 -> PWM5/1
  Demux/7 -> PWM4/1
  Demux/8 -> PWM10/1
  Demux/9 -> PWM9/1
  Demux/10 -> PWM8/1
  Demux/11 -> PWM12/1
  Demux/12 -> PWM11/1
  PWM6/1 -> Mux/1
  PWM2/1 -> Mux/2
  PWM11/1 -> Mux/12
  PWM12/1 -> Mux/11
  PWM3/1 -> Mux/3
  PWM1/1 -> Mux/4
  PWM7/1 -> Mux/5
  PWM5/1 -> Mux/6
  PWM4/1 -> Mux/7
  PWM10/1 -> Mux/8
  PWM9/1 -> Mux/9
  PWM8/1 -> Mux/10
  Mux1/1 -> Matrix Multiply/2
  Constant/1 -> Matrix Multiply/1
  Matrix Multiply/1 -> Real torque/1
  PWM18/1 -> Mux1/3
  PWM21/1 -> Mux1/1
  Demux1/2 -> PWM17/1
  PWM17/1 -> Mux1/2
  PWM13/1 -> Mux1/4
  uTimes/1 -> Demux1/1
  Demux1/1 -> PWM21/1
  Demux1/4 -> PWM13/1
  Demux1/3 -> PWM18/1

== system main/Real physics/Air drag ==
  Body attitude [Earth inertial frame] : Inport  Unit=1
  S/c position [Earth inertial frame][km] : Inport  Port=2  OutDataTypeStr=double  Unit=km  PortDimensions=3
  S/c velocity [Earth inertial frame][km/s] : Inport  Port=3  OutDataTypeStr=double  Unit=km/s
  Air density : Subsystem
  Constant : Constant  Value=Spacecraft  OutDataTypeStr=Bus: SpacecraftDT
  Constant1 : Constant  Value=Earth.equatorialRadius
  Constant2 : Constant  Value=2*pi/Earth.siderealDay
  Cross Product : vrlib/Utilities/Cross Product
  Gain : Gain  Gain=[0;0;1]
  MATLAB Function : MATLAB Function  TreatAsAtomicUnit=on
  Sum : Sum  Inputs=+-|
  Sum1 : Sum  Inputs=|-+
  Terminator : Terminator
  Vector magnitude and direction1 : SADlibrary/Vector magnitude and direction  SystemSampleTime=-1  VariantActivationTime=update diagram  Latency=0  AutoFrameSizeCalculation=off
  Vector rotate : SADlibrary/Vector rotate  SystemSampleTime=-1  VariantActivationTime=update diagram  Latency=0  AutoFrameSizeCalculation=off
  Torque [body frame][N m] : Outport  Unit=N*m
  Force [body frame][N] : Outport  Port=2  Unit=N
  wires:
  Vector magnitude and direction1/1 -> Sum/1
  Body attitude [Earth inertial frame]/1 -> Vector rotate/1
  MATLAB Function/2(T) -> Torque [body frame][N m]/1
  MATLAB Function/1(F) -> Force [body frame][N]/1
  Constant/1 -> MATLAB Function/3(Spacecraft)
  Vector rotate/1 -> MATLAB Function/2(relVel)
  Constant1/1 -> Sum/2
  Constant2/1 -> Gain/1
  Gain/1 -> Cross Product/1
  Cross Product/1 -> Sum1/1
  S/c velocity [Earth inertial frame][km/s]/1 -> Sum1/2
  Sum1/1 -> Vector rotate/2
  Sum/1 -> Air density/1(Height)
  Air density/1(Air density) -> MATLAB Function/1(rho)
  S/c position [Earth inertial frame][km]/1 -> Vector magnitude and direction1/1, Cross Product/2
  Vector magnitude and direction1/2 -> Terminator/1

== system main/Real physics/Gravity gradient (torque only) ==
  note: $3\frac{\mu}{R^3}$
  note: $\mathbf{c}$
  note: $\mathbf{R} = \text{Earth position wrt to the spacecraft$ calculated in the body reference frame
      | $R = \left|| \mathbf{R} \left||$
      | $\mathbf{c} = \frac{\mathbf{R}}{R}$
      | $\mathbf{M} = 3\frac{\mu}{R^3} \left[ (-I_y + I_z) c_y c_z \quad (-I_z + I_x) c_z c_x \quad (-I_x + I_y) c_x c_y\right]^T$
      |
      | Please note that
      | $[b \quad c \quad a] = \text{Cycle_3_vector}\left([a \quad b \quad c]\right)$
  Inertia [body frame][kg m²] : Inport  Unit=kg*m^2
  Body attitude [Earth inertial frame] : Inport  Port=2  Unit=1
  S/c position [Earth inertial frame][km] : Inport  Port=3  OutDataTypeStr=double  Unit=km
  Constant : Constant  Value=Earth.mu
  Cycle vector{,1..3} (4 alike) : SADlibrary/Cycle vector  SystemSampleTime=-1  VariantActivationTime=update diagram  Latency=0  AutoFrameSizeCalculation=off
  Divide1 : Product  Inputs=//*
  Gain1 : Gain  Gain=3
  Product : Product  Inputs=4
  Square : Math  Operator=square  SaturateOnIntegerOverflow=on
  Sum : Sum  Inputs=+-|
  Vector magnitude and direction1 : SADlibrary/Vector magnitude and direction  SystemSampleTime=-1  VariantActivationTime=update diagram  Latency=0  AutoFrameSizeCalculation=off
  Vector rotate : SADlibrary/Vector rotate  SystemSampleTime=-1  VariantActivationTime=update diagram  Latency=0  AutoFrameSizeCalculation=off
  Torque [body frame][N m] : Outport  Unit=N*m
  wires:
  Inertia [body frame][kg m²]/1 -> Cycle vector/1
  Product/1 -> Torque [body frame][N m]/1
  Constant/1 -> Gain1/1
  Divide1/1 -> Product/4
  Cycle vector3/1 -> Product/3, Cycle vector2/1
  Cycle vector/1 -> Sum/2, Cycle vector1/1
  Cycle vector2/1 -> Product/2
  Cycle vector1/1 -> Sum/1
  Sum/1 -> Product/1
  Gain1/1 -> Divide1/3
  Square/1 -> Divide1/1
  Vector magnitude and direction1/1 -> Divide1/2, Square/1
  S/c position [Earth inertial frame][km]/1 -> Vector magnitude and direction1/1
  Vector magnitude and direction1/2 -> Vector rotate/2
  Vector rotate/1 -> Cycle vector3/1
  Body attitude [Earth inertial frame]/1 -> Vector rotate/1

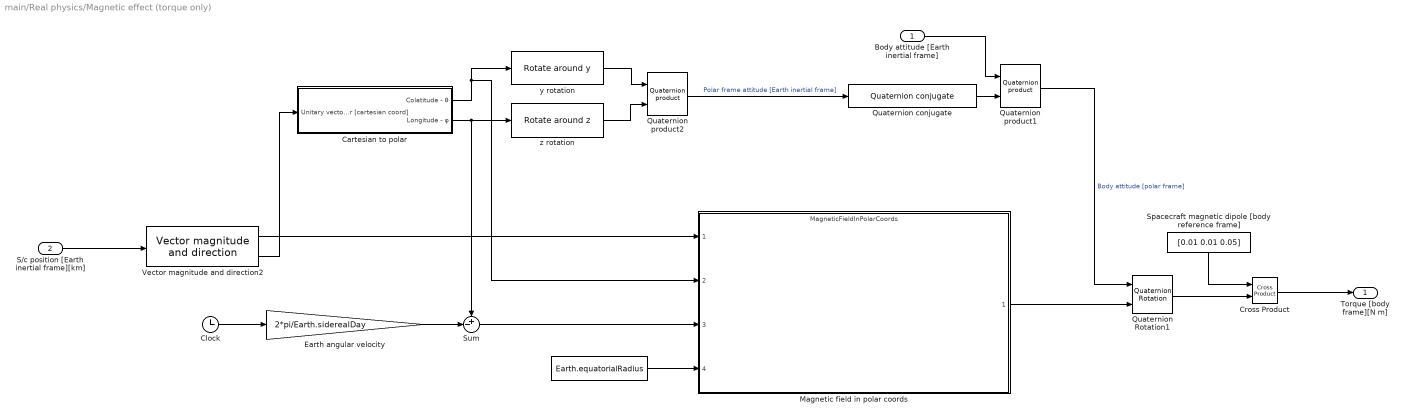
== system main/Real physics/Magnetic effect (torque only) ==
  Body attitude [Earth inertial frame] : Inport  Unit=1
  S/c position [Earth inertial frame][km] : Inport  Port=2  OutDataTypeStr=double  Unit=km
  " " : Constant  Value=Earth.equatorialRadius
  Cartesian to polar : Subsystem
  Clock : Clock
  Cross Product : vrlib/Utilities/Cross Product
  Earth angular velocity : Gain  Gain=2*pi/Earth.siderealDay
  Magnetic field in polar coords : ModelReference  ModelNameDialog=MagneticFieldInPolarCoords.slx  SimulationMode=Normal  ModelReferenceVersion=1.3
  Quaternion Rotation1 : aerolibutil/Quaternion Rotation
  Quaternion conjugate : SADlibrary/Quaternion conjugate  SystemSampleTime=-1  VariantActivationTime=update diagram  Latency=0  AutoFrameSizeCalculation=off
  Quaternion product1 : SADlibrary/Quaternion product  SystemSampleTime=-1  VariantActivationTime=update diagram  Latency=0  AutoFrameSizeCalculation=off
  Quaternion product2 : SADlibrary/Quaternion product  SystemSampleTime=-1  VariantActivationTime=update diagram  Latency=0  AutoFrameSizeCalculation=off
  Spacecraft magnetic dipole [body reference frame] : Constant  Value=[0.01 0.01 0.05]
  Sum : Sum  Inputs=+-|
  Vector magnitude and direction2 : SADlibrary/Vector magnitude and direction  SystemSampleTime=-1  VariantActivationTime=update diagram  Latency=0  AutoFrameSizeCalculation=off
  y rotation : SADlibrary/Rotate around y  SystemSampleTime=-1  VariantActivationTime=update diagram  Latency=0  AutoFrameSizeCalculation=off
  z rotation : SADlibrary/Rotate around z  SystemSampleTime=-1  VariantActivationTime=update diagram  Latency=0  AutoFrameSizeCalculation=off
  Torque [body frame][N m] : Outport  OutDataTypeStr=double  Unit=N*m
  wires:
  Cartesian to polar/2(Longitude - φ) -> z rotation/1, Sum/1
  Cartesian to polar/1(Colatitude - θ) -> y rotation/1, Magnetic field in polar coords/2
  y rotation/1 -> Quaternion product2/1
  z rotation/1 -> Quaternion product2/2
  Quaternion product2/1 -> Quaternion conjugate/1  "Polar frame attitude [Earth inertial frame]"
  Body attitude [Earth inertial frame]/1 -> Quaternion product1/1
  Quaternion conjugate/1 -> Quaternion product1/2
  Quaternion product1/1 -> Quaternion Rotation1/1  "Body attitude [polar frame]"
  Clock/1 -> Earth angular velocity/1
  Earth angular velocity/1 -> Sum/2
  Sum/1 -> Magnetic field in polar coords/3
  " "/1 -> Magnetic field in polar coords/4
  Spacecraft magnetic dipole [body reference frame]/1 -> Cross Product/1
  Quaternion Rotation1/1 -> Cross Product/2
  Cross Product/1 -> Torque [body frame][N m]/1
  Magnetic field in polar coords/1 -> Quaternion Rotation1/2
  Vector magnitude and direction2/2 -> Cartesian to polar/1(Unitary vector [cartesian coord])
  Vector magnitude and direction2/1 -> Magnetic field in polar coords/1
  S/c position [Earth inertial frame][km]/1 -> Vector magnitude and direction2/1

== system main/Real physics/Rotational dynamic ==
  Inertia [body frame][kg m²] : Inport  Unit=kg*m^2  PortDimensions=3
  External torque [body frame][N m] : Inport  Port=2  Unit=N*m  PortDimensions=3
  Constant : Constant  Value=Spacecraft.initialAngularSpeed
  Constant1 : Constant  Value=Spacecraft.initialAttitude
  "Euler equations (rigid body) " : Subsystem
  Integrator : Integrator  InitialConditionSource=external  InitialCondition=initCond
  Integrator1 : Integrator  InitialConditionSource=external
  Kinematics with quaternions : Subsystem
  Quaternion Normalize : sharedutil/Quaternion Normalize  aMode=aMode
      settings: SourceProductBaseCode=AE,PW,DR,MT,UV,VE
  Angular velocity [body frame][rad/s] : Outport  OutDataTypeStr=double  Unit=rad/s  PortDimensions=3
  Body attitude [Earth inertial frame] : Outport  Port=2  OutDataTypeStr=double  Unit=1  PortDimensions=4
  wires:
  Inertia [body frame][kg m²]/1 -> "Euler equations (rigid body) "/2(Inertia [body reference frame])
  Constant/1 -> Integrator/2
  External torque [body frame][N m]/1 -> "Euler equations (rigid body) "/3(External torque [body reference frame])
  Integrator/1 -> Kinematics with quaternions/2(omega [body frame]), Angular velocity [body frame][rad/s]/1, "Euler equations (rigid body) "/1(omega [body reference frame])
  "Euler equations (rigid body) "/1(omega dot [body reference frame]) -> Integrator/1
  Constant1/1 -> Integrator1/2
  Kinematics with quaternions/1(q dot) -> Integrator1/1
  Integrator1/1 -> Quaternion Normalize/1
  Quaternion Normalize/1 -> Kinematics with quaternions/1(q), Body attitude [Earth inertial frame]/1

== system main/Real physics/Solar radiation pressure (torque only) ==
  note: Note: I made the assumption to consider geometric body axis = to principal body axis
  Sun position wrt s/c [body frame][km] : Inport  OutDataTypeStr=double  Unit=km
  " " : Constant  Value=Spacecraft  OutDataTypeStr=Bus: SpacecraftDT
  MATLAB Function : MATLAB Function  TreatAsAtomicUnit=on
  Solar radiation pressure : Subsystem
  Vector magnitude and direction2 : SADlibrary/Vector magnitude and direction  SystemSampleTime=-1  VariantActivationTime=update diagram  Latency=0  AutoFrameSizeCalculation=off
  Force [body frame][N] : Outport  OutDataTypeStr=double  Unit=N
  Torque [body frame][N m] : Outport  Port=2  OutDataTypeStr=double  Unit=N*m
  wires:
  Vector magnitude and direction2/1 -> Solar radiation pressure/1(Distance from the sun)
  Solar radiation pressure/1(SRP) -> MATLAB Function/2(SRP)
  Vector magnitude and direction2/2 -> MATLAB Function/1(sunDir)
  " "/1 -> MATLAB Function/3(Spacecraft)
  MATLAB Function/2(T) -> Torque [body frame][N m]/1
  MATLAB Function/1(F) -> Force [body frame][N]/1
  Sun position wrt s/c [body frame][km]/1 -> Vector magnitude and direction2/1

== system main/Real physics/Sun position wrt s//c ==
  S/c position [Earth inertial frame][km] : Inport  OutDataTypeStr=double  Unit=km
  Body attitude [Earth inertial frame] : Inport  Port=2  OutDataTypeStr=double  Unit=1
  Degrees to Radians : simulink_extras/Transformations/Degrees to Radians
  Get true anomaly1 : Subsystem
  Mux : Mux  Inputs=6
  Quaternion Rotation : aerolibutil/Quaternion Rotation
  Scope : Scope
  Sum : Sum  Inputs=|+-
  Sun position wrt Earth : Subsystem
  a : Constant  Value=149.60e6
  e : Constant  Value=.0167086
  "i, Ω, ω" : Constant  Value=0
  θ - (78° = 21st March) : Constant  Value=78
  μ Sun : Constant  Value=1.3271244001e11
  Sun position wrt s/c [body frame][km] : Outport  OutDataTypeStr=double  Unit=km
  Sun position wrt s/c [Earth inertial frame][km] : Outport  Port=2
  wires:
  θ - (78° = 21st March)/1 -> Degrees to Radians/1
  e/1 -> Mux/2
  Degrees to Radians/1 -> Mux/6
  a/1 -> Mux/1
  Mux/1 -> Get true anomaly1/2(Initial keplerian elements)
  μ Sun/1 -> Get true anomaly1/1(Planetary constant)
  "i, Ω, ω"/1 -> Mux/3, Mux/5, Mux/4
  Get true anomaly1/1(Keplerian elements) -> Sun position wrt Earth/1(Keplerian elements of the Earth around the Sun)
  Sun position wrt Earth/1(Position [Earth inertial frame][km]) -> Sum/1
  S/c position [Earth inertial frame][km]/1 -> Sum/2
  Sum/1 -> Scope/1, Sun position wrt s/c [Earth inertial frame][km]/1, Quaternion Rotation/2  "Sun wrt s/c [Earth inertial frame][km]"
  Body attitude [Earth inertial frame]/1 -> Quaternion Rotation/1
  Quaternion Rotation/1 -> Sun position wrt s/c [body frame][km]/1

== system main/Real physics/Translational dynamic ==
  Initial s/c position [Earth inertial frame][km] : Inport  Unit=km
  Initial s/c velocity [Earth inertial frame][km/s] : Inport  Port=2  Unit=km/s
  Integrator : Integrator  InitialConditionSource=external  AbsoluteTolerance=1e-14
  Integrator1 : Integrator  InitialConditionSource=external  AbsoluteTolerance=1e-14
  J2 effect : Subsystem
  Main contribution : Subsystem
  Sum : Sum
  S/c position [ECI][km] : Outport  OutDataTypeStr=double  Unit=km  PortDimensions=3
  S/c velocity [ECI][kim/s] : Outport  Port=2  OutDataTypeStr=double  Unit=km/s  PortDimensions=3
  wires:
  Initial s/c velocity [Earth inertial frame][km/s]/1 -> Integrator/2
  Initial s/c position [Earth inertial frame][km]/1 -> Integrator1/2
  Integrator/1 -> S/c velocity [ECI][kim/s]/1, Integrator1/1
  Integrator1/1 -> S/c position [ECI][km]/1, Main contribution/1(Position [Earth inertial frame]), J2 effect/1(Position [Earth inertial frame])
  J2 effect/1(Acceleration [Earth inertial frame]) -> Sum/1
  Main contribution/1(Acceleration [Earth inertial frame]) -> Sum/2
  Sum/1 -> Integrator/1

== system main/Solve Whabba's problem/Angles 2 vector ==
  In1 : Inport
  Constant : Constant
  Demux : Demux  Outputs=2
  Demux1 : Demux  Outputs=3
  Divide : Product  Inputs=/*
  Mux : Mux  Inputs=3
  Sqrt : Sqrt  SaturateOnIntegerOverflow=on
  Square : Math  Operator=square  SaturateOnIntegerOverflow=on
  Sum : Sum  Inputs=+++
  Tan : Trigonometry  Operator=tan
  Out1 : Outport
  wires:
  Divide/1 -> Out1/1
  Square/1 -> Demux1/1
  Demux1/3 -> Sum/3
  Sum/1 -> Sqrt/1
  Demux/2 -> Mux/2
  Mux/1 -> Divide/2, Square/1
  Demux1/2 -> Sum/2
  In1/1 -> Tan/1
  Demux/1 -> Mux/1
  Sqrt/1 -> Divide/1
  Constant/1 -> Mux/3
  Tan/1 -> Demux/1
  Demux1/1 -> Sum/1

== system main/Solve Whabba's problem/Angles 2 vector1 ==
  Star 2 : Inport
  Constant : Constant
  Demux : Demux  Outputs=2
  Demux1 : Demux  Outputs=3
  Divide : Product  Inputs=/*
  Mux : Mux  Inputs=3
  Sqrt : Sqrt  SaturateOnIntegerOverflow=on
  Square : Math  Operator=square  SaturateOnIntegerOverflow=on
  Sum : Sum  Inputs=+++
  Tan : Trigonometry  Operator=tan
  Out1 : Outport
  wires:
  Divide/1 -> Out1/1
  Square/1 -> Demux1/1
  Demux1/3 -> Sum/3
  Sum/1 -> Sqrt/1
  Demux/2 -> Mux/2
  Mux/1 -> Divide/2, Square/1
  Demux1/2 -> Sum/2
  Star 2/1 -> Tan/1
  Demux/1 -> Mux/1
  Sqrt/1 -> Divide/1
  Constant/1 -> Mux/3
  Tan/1 -> Demux/1
  Demux1/1 -> Sum/1

== system main/Solve Whabba's problem/Angles 2 vector2 ==
  Star 3 : Inport
  Constant : Constant
  Demux : Demux  Outputs=2
  Demux1 : Demux  Outputs=3
  Divide : Product  Inputs=/*
  Mux : Mux  Inputs=3
  Sqrt : Sqrt  SaturateOnIntegerOverflow=on
  Square : Math  Operator=square  SaturateOnIntegerOverflow=on
  Sum : Sum  Inputs=+++
  Tan : Trigonometry  Operator=tan
  Out1 : Outport
  wires:
  Divide/1 -> Out1/1
  Square/1 -> Demux1/1
  Demux1/3 -> Sum/3
  Sum/1 -> Sqrt/1
  Demux/2 -> Mux/2
  Mux/1 -> Divide/2, Square/1
  Demux1/2 -> Sum/2
  Star 3/1 -> Tan/1
  Demux/1 -> Mux/1
  Sqrt/1 -> Divide/1
  Constant/1 -> Mux/3
  Tan/1 -> Demux/1
  Demux1/1 -> Sum/1
